simulink model "rl2"  (R2017b)
settings: Solver=VariableStepAuto  StartTime=0.0  StopTime=0.08  MaxStep=1e-4  RelTol=1e-3
values from neighbouring files (symbols this model uses):
  F_b = 50.0    (= 50)    [rl2_ini.m]    (also in rl_ini.m; rl_ini_jm.m; rlc_gformer_ini.m)
  L_1 = 10e-3    (= 0.01)    [rl2_ini.m]
  L_2 = 1e-3    (= 0.001)    [rl2_ini.m]
  R_1 = 1.0    (= 1)    [rl2_ini.m]
  R_2 = 1.0    (= 1)    [rl2_ini.m]
undefined symbols (not defined in the file or in its folder): T_s_power
libraries: powerlib x10, powerlib_meascontrol x7
settings Model: Creator=jmmauricio  LastModifiedBy=jmmau
settings CodeAppCC: StateflowObjectComments=on
settings SimscapeCC: SimscapeNormalizeSystem=off

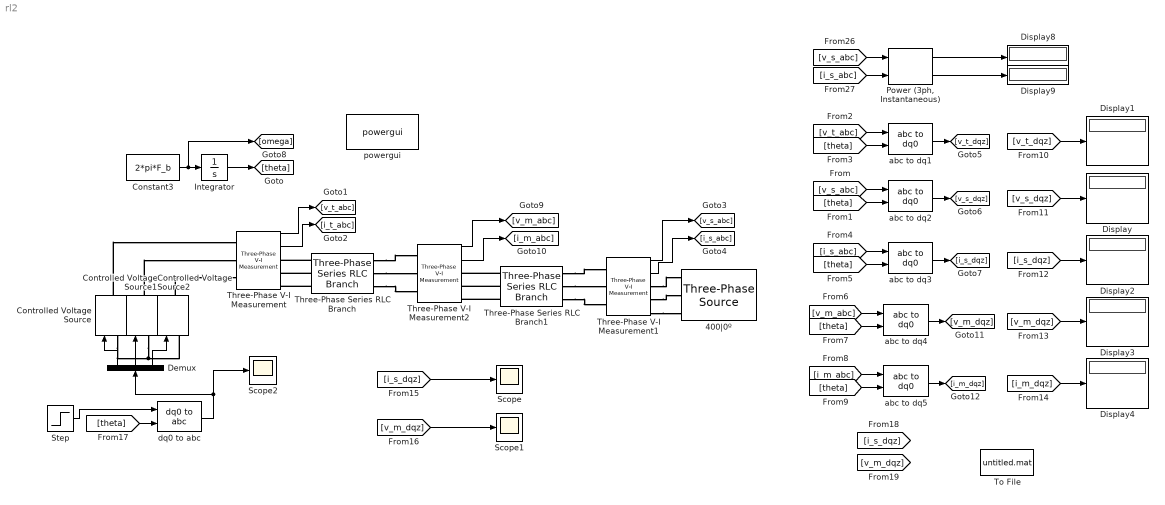
== system rl2 ==
  400|0º : powerlib/Electrical Sources/Three-Phase Source  InternalConnection=Yg  VoltagePhases=off  Voltage=400  PhaseAngle=0  Voltage_phases=[25e3 25e3 25e3]/sqrt(3)  PhaseAngles_phases=[0 -120 +120]  Frequency=50  NonIdealSource=off  SpecifyImpedance=off  Resistance=0.8929  Inductance=16.58e-3  ShortCircuitLevel=100e6  BaseVoltage=25e3  XRratio=7  BusType=swing  Pref=10e3  Qref=0  Prefabc=[10e3, 10e3, 10e3]  Qrefabc=[0, 0, 0]  Qmin=-inf  Qmax=inf
  Constant3 : Constant  Value=2*pi*F_b
  Controlled Voltage Source : powerlib/Electrical Sources/Controlled Voltage Source  Initialize=on  Source_Type=AC  Amplitude=0  Phase=0  Frequency=0  Measurements=None
  Controlled Voltage Source1 : powerlib/Electrical Sources/Controlled Voltage Source  Initialize=on  Source_Type=AC  Amplitude=0  Phase=0  Frequency=0  Measurements=None
  Controlled Voltage Source2 : powerlib/Electrical Sources/Controlled Voltage Source  Initialize=on  Source_Type=AC  Amplitude=0  Phase=0  Frequency=0  Measurements=None
  Demux : Demux  Outputs=3
  Display{,1..4,8..9} (7 alike) : Display
  Integrator : Integrator
  "Power (3ph, Instantaneous)" : powerlib_meascontrol/Measurements/Power (3ph, Instantaneous)
      settings: SourceProductName=Simscape Power Systems
  Scope : Scope
  Scope1 : Scope
  Scope2 : Scope
  Step : Step  Time=0.02  Before=[0,-400*sqrt(2/3),0]  After=[50,-400*sqrt(2/3),0]  SampleTime=0
  Three-Phase Series RLC Branch : powerlib/Elements/Three-Phase Series RLC Branch  LConnTagsString=A|B|C  RConnTagsString=A|B|C  BranchType=RL  Resistance=R_1  Inductance=L_1  Capacitance=1e-6  Measurements=None
  Three-Phase Series RLC Branch1 : powerlib/Elements/Three-Phase Series RLC Branch  LConnTagsString=A|B|C  RConnTagsString=A|B|C  BranchType=RL  Resistance=R_2  Inductance=L_2  Capacitance=1e-6  Measurements=None
  Three-Phase V-I Measurement : powerlib/Measurements/Three-Phase V-I Measurement  VoltageMeasurement=phase-to-ground  SetLabelV=off  LabelV=Vabc  Vpu=off  VpuLL=off  CurrentMeasurement=yes  SetLabelI=off  LabelI=Iabc  Ipu=off  Pbase=100e6  Vbase=500e3  OutputType=Complex  PhasorSimulation=off  PSBequivalent=0
  Three-Phase V-I Measurement1 : powerlib/Measurements/Three-Phase V-I Measurement  VoltageMeasurement=phase-to-ground  SetLabelV=off  LabelV=Vabc  Vpu=off  VpuLL=off  CurrentMeasurement=yes  SetLabelI=off  LabelI=Iabc  Ipu=off  Pbase=100e6  Vbase=500e3  OutputType=Complex  PhasorSimulation=off  PSBequivalent=0
  Three-Phase V-I Measurement2 : powerlib/Measurements/Three-Phase V-I Measurement  VoltageMeasurement=phase-to-ground  SetLabelV=off  LabelV=Vabc  Vpu=off  VpuLL=off  CurrentMeasurement=yes  SetLabelI=off  LabelI=Iabc  Ipu=off  Pbase=100e6  Vbase=500e3  OutputType=Complex  PhasorSimulation=off  PSBequivalent=0
  To File : ToFile  SaveFormat=Timeseries
  abc to dq{1..5} (5 alike) : powerlib_meascontrol/Transformations/abc to dq0  Alignment=Aligned with phase A axis
  dq0 to abc : powerlib_meascontrol/Transformations/dq0 to abc  Alignment=Aligned with phase A axis
  powergui : powerlib/powergui  Priority=1  SimulationMode=Continuous  SampleTime=T_s_power  frequency=60  Iterations=50  frequencyindice=50  Pbase=100e6  ErrMax=1e-4  UnitsV=kV  UnitsW=MW  buscounter=0  FunctionMessages=off  echomessages=off  EnableUseOfTLC=off  CurrentSourceSwitches=off  DisableSnubberDevices=off  DisableRonSwitches=off  DisableVfSwitches=off  DisplayEquations=off  SolverType=Tustin/Backward Euler (TBE)  Interpol=off  ExternalGateDelay=off  methode=off  Ts=100  x0status=zero  SPID=on  SwTol=0  HookPort=off  RestoreLinks=warning  ResistiveCurrentMeasurement=off  Frange=[0:2:500]  Ylog=off  Xlog=on  ShowGrid=off  save=off  variable=ZData  structure=0  ZoomFFT=off  StartTime=0.0  cycles=1  DisplayStyle=1  fundamental=60  FreqAxis=off  MaxFrequency=1000  frequencyindicesteady=1  RmsSteady=1  display=off
  wires:
  Constant3/1 -> [omega], Integrator/1
  Integrator/1 -> [theta]
  Three-Phase V-I Measurement/1 -> [v_t_abc]
  Three-Phase V-I Measurement/2 -> [i_t_abc]
  Three-Phase V-I Measurement1/2 -> [i_s_abc]
  Three-Phase V-I Measurement1/1 -> [v_s_abc]
  [v_s_abc] -> abc to dq2/1
  [theta] -> abc to dq2/2
  [v_t_abc] -> abc to dq1/1
  [theta] -> abc to dq1/2
  [i_s_abc] -> abc to dq3/1
  [theta] -> abc to dq3/2
  abc to dq1/1 -> [v_t_dqz]
  abc to dq2/1 -> [v_s_dqz]
  abc to dq3/1 -> [i_s_dqz]
  [v_t_dqz] -> Display1/1
  [v_s_dqz] -> Display/1
  [i_s_dqz] -> Display2/1
  [v_s_abc] -> "Power (3ph, Instantaneous)"/1
  [i_s_abc] -> "Power (3ph, Instantaneous)"/2
  "Power (3ph, Instantaneous)"/2 -> Display9/1
  "Power (3ph, Instantaneous)"/1 -> Display8/1
  Three-Phase V-I Measurement2/2 -> [i_m_abc]
  Three-Phase V-I Measurement2/1 -> [v_m_abc]
  abc to dq4/1 -> [v_m_dqz]
  abc to dq5/1 -> [i_m_dqz]
  [theta] -> abc to dq5/2
  [v_m_abc] -> abc to dq4/1
  [i_m_abc] -> abc to dq5/1
  [theta] -> abc to dq4/2
  [v_m_dqz] -> Display3/1
  [i_m_dqz] -> Display4/1
  [i_s_dqz] -> Scope/1
  [v_m_dqz] -> Scope1/1
  Demux/3 -> Controlled Voltage Source2/1
  Demux/2 -> Controlled Voltage Source1/1
  Demux/1 -> Controlled Voltage Source/1
  dq0 to abc/1 -> Scope2/1, Demux/1
  [theta] -> dq0 to abc/2
  Step/1 -> dq0 to abc/1
  connections:
  Controlled Voltage Source/RConn1 -- Three-Phase V-I Measurement/LConn1
  Controlled Voltage Source1/RConn1 -- Three-Phase V-I Measurement/LConn2
  Controlled Voltage Source2/RConn1 -- Three-Phase V-I Measurement/LConn3
  Three-Phase Series RLC Branch/LConn1 -- Three-Phase V-I Measurement/RConn1
  Three-Phase Series RLC Branch/LConn2 -- Three-Phase V-I Measurement/RConn2
  Three-Phase Series RLC Branch/LConn3 -- Three-Phase V-I Measurement/RConn3
  Three-Phase V-I Measurement1/RConn3 -- 400|0º/RConn3
  Three-Phase V-I Measurement1/RConn2 -- 400|0º/RConn2
  Three-Phase V-I Measurement1/RConn1 -- 400|0º/RConn1
  Three-Phase Series RLC Branch/RConn1 -- Three-Phase V-I Measurement2/LConn1
  Three-Phase Series RLC Branch/RConn2 -- Three-Phase V-I Measurement2/LConn2
  Three-Phase Series RLC Branch/RConn3 -- Three-Phase V-I Measurement2/LConn3
  Controlled Voltage Source/LConn1 -- Controlled Voltage Source1/LConn1 -- Controlled Voltage Source2/LConn1
  Three-Phase Series RLC Branch1/LConn2 -- Three-Phase V-I Measurement2/RConn2
  Three-Phase Series RLC Branch1/LConn3 -- Three-Phase V-I Measurement2/RConn3
  Three-Phase Series RLC Branch1/LConn1 -- Three-Phase V-I Measurement2/RConn1
  Three-Phase Series RLC Branch1/RConn1 -- Three-Phase V-I Measurement1/LConn1
  Three-Phase Series RLC Branch1/RConn2 -- Three-Phase V-I Measurement1/LConn2
  Three-Phase Series RLC Branch1/RConn3 -- Three-Phase V-I Measurement1/LConn3
